simulink model "TDS_TF_varyingTH2"  (R2019b)
settings: Solver=VariableStepAuto  StartTime=0.0  StopTime=1000  RelTol=1e-3
values from neighbouring files (symbols this model uses):
  tau1 = 15    [SmithControl.m]    (also in TimeDelayParameters.m; positivity_matrix.m)
  tau2 = 20    [SmithControl.m]    (also in TimeDelayParameters.m = 30; positivity_matrix.m = 30)
  th1 = 0.85    [AP_TimeDelay.m]    (also in SmithControl.m; TimeDelayParameters.m = 0.32; positivity_matrix.m; rscale.m)
  th2 = 50    [AP_TimeDelay.m]    (also in SmithControl.m; TimeDelayParameters.m; positivity_matrix.m; rscale.m)
  th3 = 60    [AP_TimeDelay.m]    (also in SmithControl.m; TimeDelayParameters.m = 70; positivity_matrix.m; rscale.m)
  th4 = 5    [AP_TimeDelay.m]    (also in SmithControl.m; TimeDelayParameters.m = 2.7; positivity_matrix.m; rscale.m)
  th5 = 20    [AP_TimeDelay.m]    (also in SmithControl.m; TimeDelayParameters.m = 22; positivity_matrix.m; rscale.m)
settings Model: Creator=akshita_jain  LastModifiedBy=akshita_jain

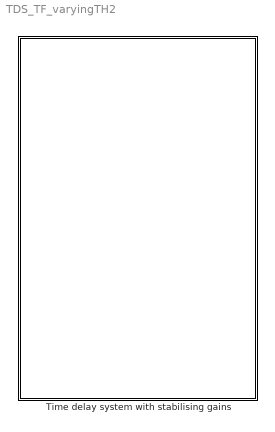
== system TDS_TF_varyingTH2 ==
  Time delay system with stabilising gains : Subsystem

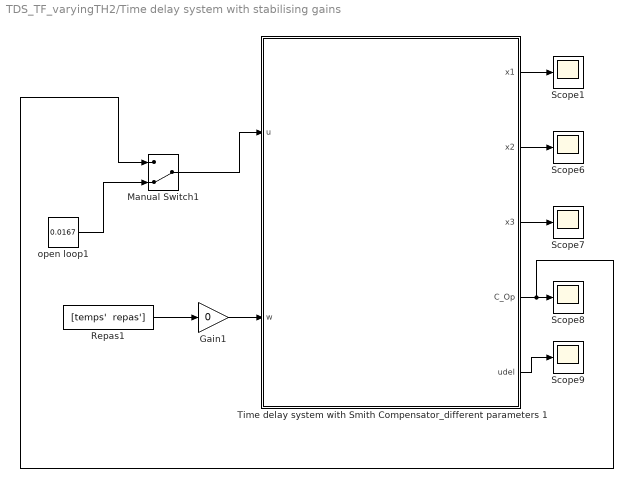
== system TDS_TF_varyingTH2/Time delay system with stabilising gains ==
  Gain1 : Gain  Gain=0
  Manual Switch1 : ManualSwitch  CurrentSetting=0
  Repas1 : FromWorkspace  VariableName="[temps'  repas']"  SampleTime=0
  Scope{1,6..9} (5 alike) : Scope
  Time delay system with Smith Compensator_different parameters 1 : Subsystem
  open loop1 : Constant  Value=0.0167
  wires:
  Manual Switch1/1 -> Time delay system with Smith Compensator_different parameters 1/1(u)
  Gain1/1 -> Time delay system with Smith Compensator_different parameters 1/2(w)
  Time delay system with Smith Compensator_different parameters 1/3(x3) -> Scope7/1
  Time delay system with Smith Compensator_different parameters 1/2(x2) -> Scope6/1
  Time delay system with Smith Compensator_different parameters 1/5(udel) -> Scope9/1
  Time delay system with Smith Compensator_different parameters 1/4(C_Op) -> Manual Switch1/1, Scope8/1
  Time delay system with Smith Compensator_different parameters 1/1(x1) -> Scope1/1
  Repas1/1 -> Gain1/1
  open loop1/1 -> Manual Switch1/2

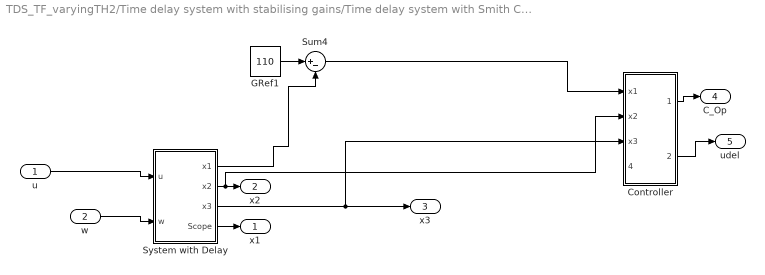
== system TDS_TF_varyingTH2/Time delay system with stabilising gains/Time delay system with Smith Compensator_different parameters 1 ==
  u : Inport
  w : Inport  Port=2
  "Controller " : Subsystem
  GRef1 : Constant  Value=110
  Sum4 : Sum  Inputs=|+-
  System with Delay : Subsystem
  x1 : Outport
  x2 : Outport  Port=2
  x3 : Outport  Port=3
  C_Op : Outport  Port=4
  udel : Outport  Port=5
  wires:
  u/1 -> System with Delay/1(u)
  w/1 -> System with Delay/2(w)
  System with Delay/4(Scope) -> x1/1
  System with Delay/1(x1) -> Sum4/2
  System with Delay/2(x2) -> "Controller "/2(x2), x2/1
  System with Delay/3(x3) -> "Controller "/3(x3), x3/1
  "Controller "/1(C_OP) -> C_Op/1
  "Controller "/2(udel) -> udel/1
  GRef1/1 -> Sum4/1
  Sum4/1 -> "Controller "/1(x1)

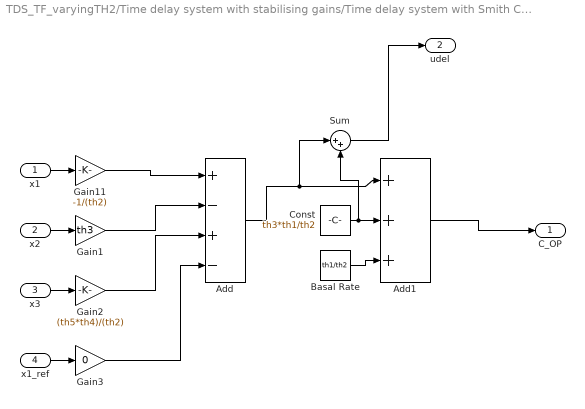
== system TDS_TF_varyingTH2/Time delay system with stabilising gains/Time delay system with Smith Compensator_different parameters 1/Controller  ==
  x1 : Inport
  x2 : Inport  Port=2
  x3 : Inport  Port=3
  x1_ref : Inport  Port=4
  Add : Sum  Inputs=+-+-
  Add1 : Sum  Inputs=+++
  Basal Rate : Constant  Value=th1/th2  VectorParams1D=off
  Const : Constant  Value=th3*th1/th2  VectorParams1D=off
  Gain1 : Gain  Gain=th3
  Gain11 : Gain  Gain=-1/(th2)
  Gain2 : Gain  Gain=(th5*th4)/(th2)
  Gain3 : Gain  Gain=0
  Sum : Sum  Inputs=|++
  C_OP : Outport
  udel : Outport  Port=2
  wires:
  x1/1 -> Gain11/1
  x2/1 -> Gain1/1
  x3/1 -> Gain2/1
  Gain11/1 -> Add/1
  Gain1/1 -> Add/2
  Gain2/1 -> Add/3
  Add/1 -> Sum/1, Add1/1
  Const/1 -> Add1/2, Sum/2
  Basal Rate/1 -> Add1/3
  Add1/1 -> C_OP/1
  Sum/1 -> udel/1
  x1_ref/1 -> Gain3/1
  Gain3/1 -> Add/4

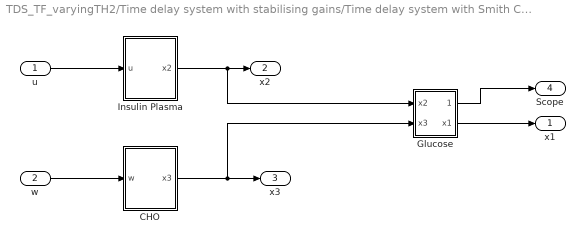
== system TDS_TF_varyingTH2/Time delay system with stabilising gains/Time delay system with Smith Compensator_different parameters 1/System with Delay ==
  u : Inport
  w : Inport  Port=2
  CHO : Subsystem
  Glucose : Subsystem
  Insulin Plasma : Subsystem
  x1 : Outport
  x2 : Outport  Port=2
  x3 : Outport  Port=3
  Scope : Outport  Port=4
  wires:
  Glucose/1(Out1) -> Scope/1
  Glucose/2(x1) -> x1/1
  w/1 -> CHO/1(w)
  Insulin Plasma/1(x2) -> x2/1, Glucose/1(x2)
  CHO/1(x3) -> x3/1, Glucose/2(x3)
  u/1 -> Insulin Plasma/1(u)

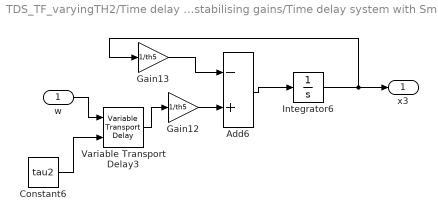
== system TDS_TF_varyingTH2/Time delay system with stabilising gains/Time delay system with Smith Compensator_different parameters 1/System with Delay/CHO ==
  w : Inport
  Add6 : Sum  Inputs=-+
  Constant6 : Constant  Value=tau2  VectorParams1D=off
  Gain12 : Gain  Gain=1/th5
  Gain13 : Gain  Gain=1/th5
  Integrator6 : Integrator  InitialCondition=0.00000000000001  ZeroCross=off
  Variable Transport Delay3 : VariableTransportDelay  VariableDelayType=Variable transport delay  MaximumDelay=35  InitialOutput=0.0000000001
  x3 : Outport
  wires:
  Integrator6/1 -> x3/1, Gain13/1
  Add6/1 -> Integrator6/1
  Constant6/1 -> Variable Transport Delay3/2
  Gain13/1 -> Add6/1
  Gain12/1 -> Add6/2
  w/1 -> Variable Transport Delay3/1
  Variable Transport Delay3/1 -> Gain12/1

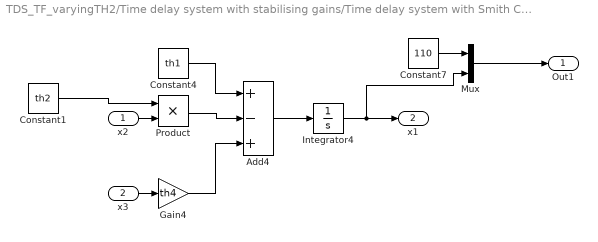
== system TDS_TF_varyingTH2/Time delay system with stabilising gains/Time delay system with Smith Compensator_different parameters 1/System with Delay/Glucose ==
  x2 : Inport
  x3 : Inport  Port=2
  Add4 : Sum  Inputs=+-+
  Constant1 : Constant  Value=th2  VectorParams1D=off
  Constant4 : Constant  Value=th1  VectorParams1D=off
  Constant7 : Constant  Value=110  VectorParams1D=off
  Gain4 : Gain  Gain=th4
  Integrator4 : Integrator  InitialCondition=110  ZeroCross=off
  Mux : Mux  Inputs=2
  Product : Product
  Out1 : Outport
  x1 : Outport  Port=2
  wires:
  x3/1 -> Gain4/1
  x2/1 -> Product/2
  Mux/1 -> Out1/1
  Add4/1 -> Integrator4/1
  Constant4/1 -> Add4/1
  Integrator4/1 -> x1/1, Mux/2
  Gain4/1 -> Add4/3
  Constant7/1 -> Mux/1
  Product/1 -> Add4/2
  Constant1/1 -> Product/1

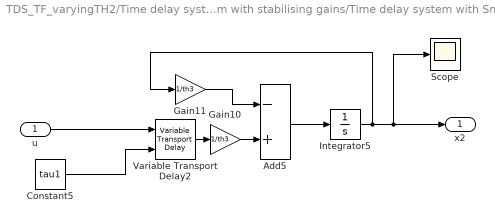
== system TDS_TF_varyingTH2/Time delay system with stabilising gains/Time delay system with Smith Compensator_different parameters 1/System with Delay/Insulin Plasma ==
  u : Inport
  Add5 : Sum  Inputs=-+
  Constant5 : Constant  Value=tau1
  Gain10 : Gain  Gain=1/th3
  Gain11 : Gain  Gain=1/th3
  Integrator5 : Integrator  InitialCondition=th1/th2  ZeroCross=off
  Scope : Scope
  Variable Transport Delay2 : VariableTransportDelay  VariableDelayType=Variable transport delay  MaximumDelay=20  InitialOutput=th1/th2
  x2 : Outport
  wires:
  Add5/1 -> Integrator5/1
  Gain11/1 -> Add5/1
  Gain10/1 -> Add5/2
  Constant5/1 -> Variable Transport Delay2/2
  Integrator5/1 -> Scope/1, x2/1, Gain11/1
  u/1 -> Variable Transport Delay2/1
  Variable Transport Delay2/1 -> Gain10/1
